simulink model "RW_withexternalT"  (R2023a)
settings: Solver=VariableStepAuto  StartTime=0.0  StopTime=50  RelTol=1e-3
libraries: slpidlib x1
settings Model: Creator=alpercakir  LastModifiedBy=alpercakir

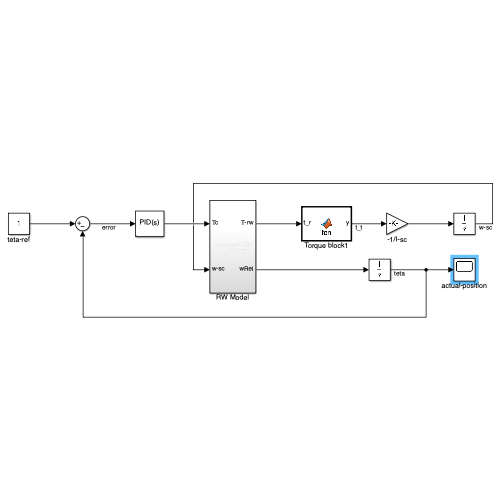
[thumbnail: Simulink's stored preview of the top-level diagram]
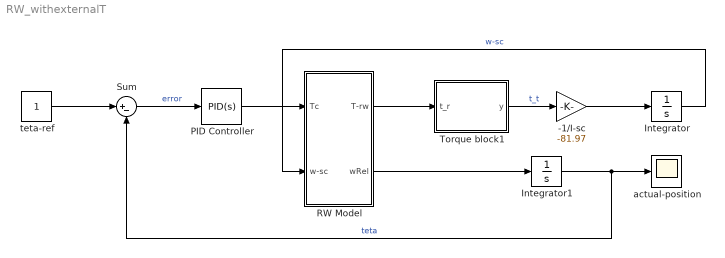
== system RW_withexternalT ==
  -1/I-sc : Gain  Gain=-81.97
  Integrator : Integrator
  Integrator1 : Integrator
  PID Controller : slpidlib/PID Controller  Controller=PID  Form=Parallel  TimeDomain=Continuous-time  UseExternalTs=off  SampleTime=-1  IntegratorMethod=Forward Euler  FilterMethod=Forward Euler  ControllerParametersSource=internal  P=0.01  I=0.01  UseKiTs=off  D=0.0025  N=100  UseFilter=on  TunerSelectOption=Transfer Function Based (PID Tuner App)  InitialConditionSource=internal  InitialConditionForIntegrator=0  InitialConditionForFilter=0  DifferentiatorICPrevScaledInput=0  ExternalReset=none  TrackingMode=off  Kt=1  LimitOutput=off  SatLimitsSource=internal  UpperSaturationLimit=inf  LowerSaturationLimit=-inf  LinearizeAsGain=on  AntiWindupMode=none  Kb=1  LimitIntegrator=off  UpperIntegratorSaturationLimit=inf  LowerIntegratorSaturationLimit=-inf  POutMin=[]  POutMax=[]  IOutMin=[]  IOutMax=[]  DOutMin=[]  DOutMax=[]  NOutMin=[]  NOutMax=[]  SumOutMin=[]  SumOutMax=[]  SaturationOutMin=[]  SaturationOutMax=[]  PParamMin=[]  PParamMax=[]  IParamMin=[]  IParamMax=[]  DParamMin=[]  DParamMax=[]  NParamMin=[]  NParamMax=[]  KbParamMin=[]  KbParamMax=[]  KtParamMin=[]  KtParamMax=[]  KbOutMin=[]  KbOutMax=[]  KtOutMin=[]  KtOutMax=[]  IntegratorOutMin=[]  IntegratorOutMax=[]  FilterOutMin=[]  FilterOutMax=[]  SumI1OutMin=[]  SumI1OutMax=[]  SumI2OutMin=[]  SumI2OutMax=[]  SumI3OutMin=[]  SumI3OutMax=[]  SumI4OutMin=[]  SumI4OutMax=[]  SumDOutMin=[]  SumDOutMax=[]  DifferentiatorOutMin=[]  DifferentiatorOutMax=[]  FilterDiffOutCoefMin=[]  FilterDiffOutCoefMax=[]  ReciprocalOutMin=[]  ReciprocalOutMax=[]  SumDenOutMin=[]  SumDenOutMax=[]  SumNumOutMin=[]  SumNumOutMax=[]  DivideOutMin=[]  DivideOutMax=[]  UdiffTsProdOutMin=[]  UdiffTsProdOutMax=[]  NTsProdOutMin=[]  NTsProdOutMax=[]  UintegralTsProdOutMin=[]  UintegralTsProdOutMax=[]  UngainTsProdOutMin=[]  UngainTsProdOutMax=[]  ClampingZeroOutDataTypeStr=Inherit: Inherit via back propagation  ClampingZeroOutMin=[]  ClampingZeroOutMax=[]  FilterDenConstantOutDataTypeStr=Inherit: Inherit via back propagation  FilterDenConstantOutMin=[]  FilterDenConstantOutMax=[]  PCopyOutDataTypeStr=Inherit: Inherit via back propagation  PCopyOutMin=[]  PCopyOutMax=[]  NCopyOutDataTypeStr=Inherit: Inherit via back propagation  NCopyOutMin=[]  NCopyOutMax=[]  IntegratorContinuousStateAttributes=''  IntegratorStateMustResolveToSignalObject=off  IntegratorRTWStateStorageClass=Auto  FilterContinuousStateAttributes=''  FilterStateMustResolveToSignalObject=off  FilterRTWStateStorageClass=Auto  ParallelPVariant=InternalParameters  IdealPVariant=Disabled  IVariant=InternalParameters  DVariant=InternalParameters  IntegratorVariant=Continuous  SatVariant=Disabled  AWVariant=Passthrough  PCopyVariant=Disabled  TRVariant=Disabled  FdbkBlocksVariant=Forward  IdealPFdbkVariant=Disabled  SatFdbkVariant=Disabled  DerivativeFilterVariant=ContFilter  NVariant=InternalParameters  NCopyVariant=Disabled  FilterICVariant=InternalICsFilter  IntegratorICVariant=InternalICs  ExternalResetVariant=Disabled  TRSumVariant=Passthrough  SumFdbkVariant=Disabled  SumVariant=Sum_PID  TsampFilterVariant=InternalTs  TsampNgainVariant=Passthrough  TsampIntegralVariant=Disabled_SignalSpec  ExternalSaturationOutDataTypeStr=Inherit: Same as second input
  RW Model : Subsystem
  Sum : Sum  Inputs=|+-
  Torque block1 : MATLAB Function  TreatAsAtomicUnit=on
  actual-position : Scope
  teta-ref : Constant
  wires:
  teta-ref/1 -> Sum/1
  -1/I-sc/1 -> Integrator/1
  PID Controller/1 -> RW Model/1(Tc)
  Sum/1 -> PID Controller/1  "error"
  Integrator1/1 -> actual-position/1, Sum/2  "teta"
  RW Model/2(wRel) -> Integrator1/1
  RW Model/1(T-rw) -> Torque block1/1(t_r)
  Torque block1/1(y) -> -1/I-sc/1  "t_t"
  Integrator/1 -> RW Model/2(w-sc)  "w-sc"

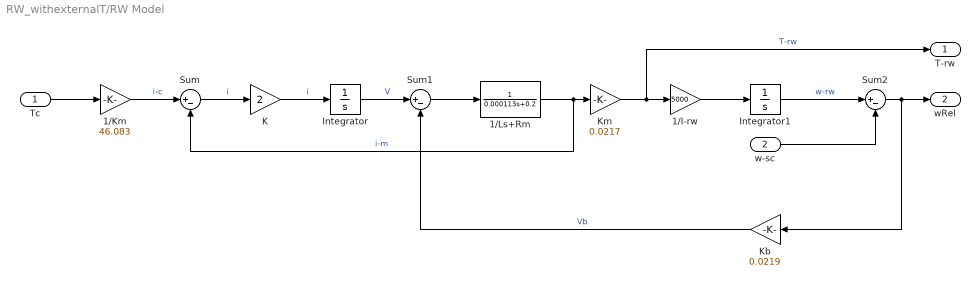
== system RW_withexternalT/RW Model ==
  Tc : Inport
  w-sc : Inport  Port=2
  1/I-rw : Gain  Gain=5000
  1/Km : Gain  Gain=46.083
  1/Ls+Rm : TransferFcn  Denominator=[0.000113 0.2]
  Integrator : Integrator
  Integrator1 : Integrator
  K : Gain  Gain=2
  Kb : Gain  Gain=0.0219
  Km : Gain  Gain=0.0217
  Sum : Sum  Inputs=|+-
  Sum1 : Sum  Inputs=|+-
  Sum2 : Sum  Inputs=|+-
  T-rw : Outport
  wRel : Outport  Port=2
  wires:
  Tc/1 -> 1/Km/1
  1/Km/1 -> Sum/1  "i-c"
  Sum/1 -> K/1  "i"
  K/1 -> Integrator/1  "i"
  Integrator/1 -> Sum1/1  "V"
  Sum1/1 -> 1/Ls+Rm/1
  1/Ls+Rm/1 -> Sum/2, Km/1  "i-m"
  Km/1 -> T-rw/1, 1/I-rw/1  "T-rw"
  1/I-rw/1 -> Integrator1/1
  Integrator1/1 -> Sum2/1  "w-rw"
  Sum2/1 -> Kb/1, wRel/1
  w-sc/1 -> Sum2/2
  Kb/1 -> Sum1/2  "Vb"

== matlab function RW_withexternalT/Torque block1 ==
  data: t_r input; y output
function y = fcn(t_r)

% constants;
q = 3*10^-12;
A = 0.0225; 
Cd = 2.2;
V=7667.8;
r=0.05;

coder.extrinsic("tf");
t_aero = 0.5*q*Cd*A*V*V*r; 
% t_gravity = ((3*M)/(2*R*R*R))*abs(I_z-I_y)
t_d = t_aero; % + t_gravity; 
t_t = t_r - t_d; % total torque equals the difference of the reaction torque and disturbance torques

y = t_t;
